simulink model "FEEDER_MODEL"  (R2024b)
settings: Solver=ode23t  StartTime=0.0  StopTime=2.4  RelTol=1e-3
libraries: spsFirstOrderFilterLib x42, spsThreePhaseVIMeasurementLib x7, spsThreePhaseDynamicLoadLib x4, spsDistributedParametersLineLib x4, spsPower3phInstantaneousLib x3, spsThreePhaseSourceLib x2, spsThreePhaseTransformerTwoWindingsLib x2, spspowerguiLib x1
(part 1 of 2)
settings Model: Creator=Baymax  LastModifiedBy=Baymax

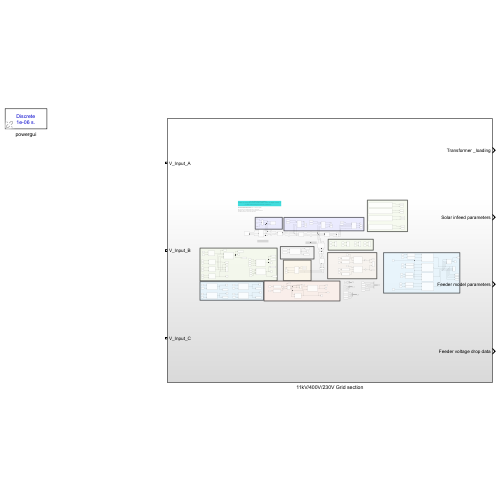
[thumbnail: Simulink's stored preview of the top-level diagram]
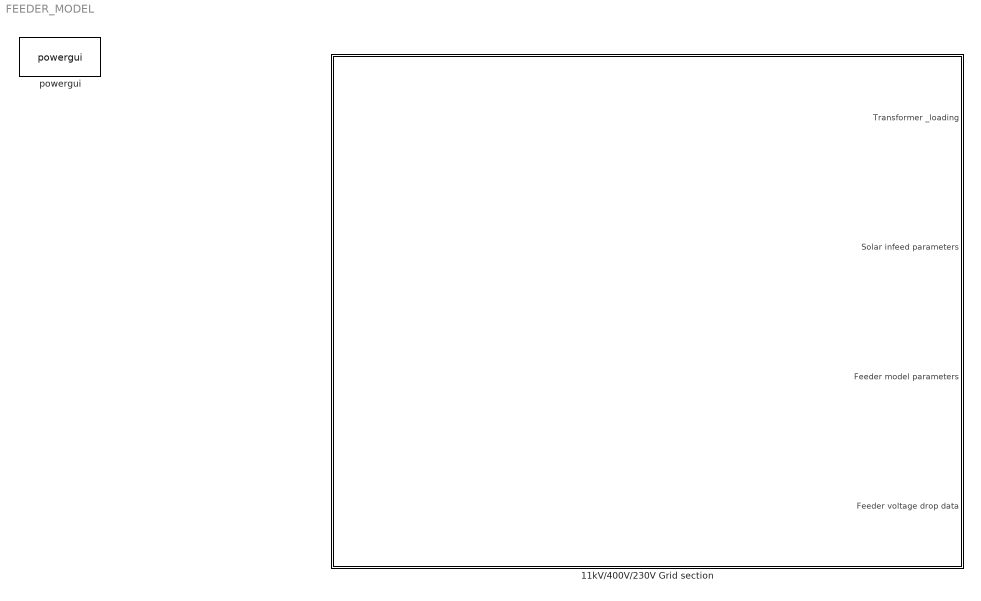
== system FEEDER_MODEL ==
  11kV/400V/230V Grid section : Subsystem
  powergui : spspowerguiLib/powergui  Priority=1  SimulationMode=Discrete  SampleTime=1e-6  frequency=60  Iterations=50  frequencyindice=50  Pbase=100e6  ErrMax=1e-4  UnitsV=kV  UnitsW=kW  buscounter=0  FunctionMessages=off  echomessages=off  EnableUseOfTLC=off  CurrentSourceSwitches=off  DisableSnubberDevices=off  DisableRonSwitches=off  DisableVfSwitches=off  DisplayEquations=off  AutomaticDiscreteSolvers=off  SolverType=Tustin/Backward Euler (TBE)  Interpol=off  ExternalGateDelay=off  methode=off  Ts=100  x0status=blocks  SPID=on  SwTol=0  HookPort=off  NonlinearTolerance=1e-4  nMaxIteration=100  ContinueOnMaxIteration=off  RestoreLinks=warning  ResistiveCurrentMeasurement=off  Frange=[0:2:500]  Ylog=off  Xlog=on  ShowGrid=off  save=off  variable=ZData  structure=0  ZoomFFT=off  StartTime=0.0  cycles=1  DisplayStyle=1  fundamental=60  FreqAxis=off  MaxFrequency=1000  frequencyindicesteady=1  RmsSteady=1  display=off

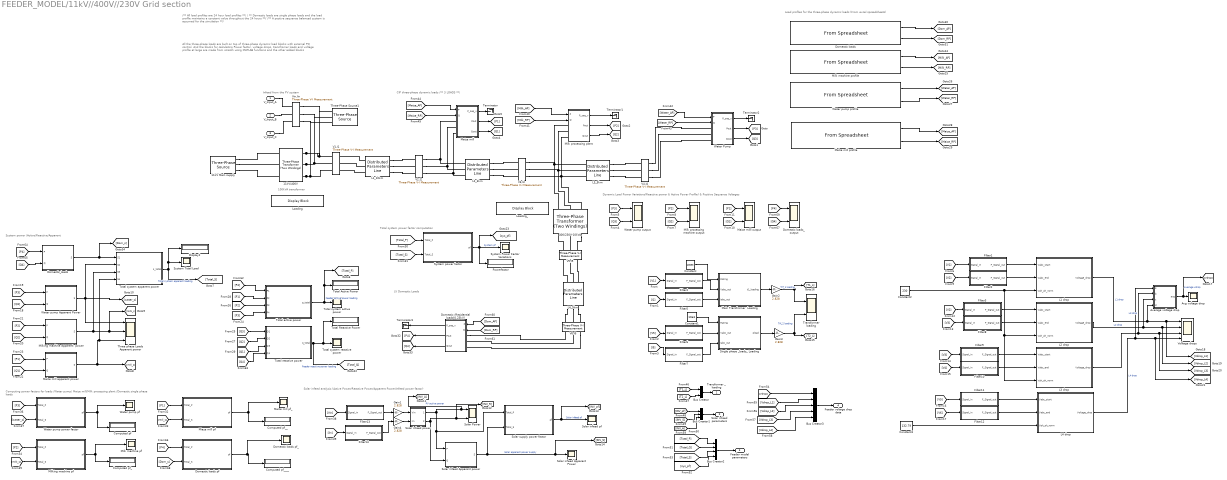
== system FEEDER_MODEL/11kV//400V//230V Grid section ==
  note: 100kVA transformer
  note: All the three-phase loads are built on top of three-phase dynamic load blocks with external PQ control.
      |
      | And the blocks for calculating Power factor, voltage drops, transfromer loads and voltage profile at large are made from scratch using MATLAB functions and the other added blocks
  note: LV Domestic Loads
  note: CIP three-phase dynamic loads /** 3 LOADS **/
  note: Solar infeed analysis (Active Power/Reactive Power/Apparent Power/Infeed power factor)
  note: Dynamic Load Power Variations(Reactive power & Active Power Profile) & Positive Sequence Voltages
  note: Computing power factors for loads /Water pump/ Maize mill/Milk processing plant /Domestic single phase loads
  note: System power /Acitve/Reactive/Apparent
  note: /** All load profiles are 24 hour load profiles **/
      |
      | / ** Domestic loads are single phase loads and the load profile maintains a constant value throughout the 24 hours **/
      |
      | /** A postive sequence balanced system is assumed for the simulation **/
  note: Load profiles for the three-phase dynamic loads (From excel spreadsheets)
  note: Total system power factor computation
  note: Infeed from the PV system
  11kV Main supply : spsThreePhaseSourceLib/Three-Phase Source  InternalConnection=Yg  VoltagePhases=off  Voltage=11e3  PhaseAngle=0  Voltage_phases=[25e3 25e3 25e3]/sqrt(3)  PhaseAngles_phases=[0 -120 +120]  Frequency=50  NonIdealSource=on  SpecifyImpedance=off  Resistance=0.8929  Inductance=16.58e-3  ShortCircuitLevel=100e6  BaseVoltage=25e3  XRratio=7  BusType=swing  Pref=10e3  Qref=0  Prefabc=[10e3, 10e3, 10e3]  Qrefabc=[0, 0, 0]  Qmin=-inf  Qmax=inf
  "11kV/400V " : spsThreePhaseTransformerTwoWindingsLib/Three-Phase Transformer (Two Windings)  Winding1Connection=Yg  Winding2Connection=Yg  CoreType=Three single-phase transformers  SetSaturation=off  Hysteresis=off  DataFile='hysteresis'  SetInitialFlux=off  Measurements=None  UNITS=pu  NominalPower=[ 100e3 , 50 ]  Winding1=[ 11e3 , 0.002 , 0.08 ]  Winding2=[ 400 , 0.002 , 0.08 ]  Rm=500  Lm=500  L0=0.5  Saturation=[ 0,0 ; 0.0024,1.2 ; 1.0,1.52 ]  InitialFluxes=[ 0.8 , -0.8 , 0.7 ]  BreakLoop=off  DiscreteSolver=Trapezoidal iterative  DataType=off  TransfoNumber=1
  "400/230V-10kVA " : spsThreePhaseTransformerTwoWindingsLib/Three-Phase Transformer (Two Windings)  Winding1Connection=Yg  Winding2Connection=Yg  CoreType=Three single-phase transformers  SetSaturation=off  Hysteresis=off  DataFile='hysteresis'  SetInitialFlux=off  Measurements=None  UNITS=pu  NominalPower=[ 10e3 , 50 ]  Winding1=[ 400 , 0.002 , 0.08 ]  Winding2=[ 230 , 0.002 , 0.08 ]  Rm=500  Lm=500  L0=0.5  Saturation=[ 0,0 ; 0.0024,1.2 ; 1.0,1.52 ]  InitialFluxes=[ 0.8 , -0.8 , 0.7 ]  BreakLoop=off  DiscreteSolver=Trapezoidal iterative  DataType=off  TransfoNumber=1
  Average voltage drop : MATLAB Function  TreatAsAtomicUnit=on
  Avg voltage drop : Scope
  Bus Creator : BusCreator  Inputs=2
  Bus Creator1 : BusCreator  Inputs=3
  Bus Creator2 : BusCreator  Inputs=4
  Bus Creator3 : BusCreator  Inputs=5
  Computed pf : Display
  Computed pf_ : Display
  Computed pf__ : Display
  Computed pf____ : Display
  Constant : Constant  Value=100e3
  Constant1 : Constant  Value=10e3
  Constant2 : Constant  Value=230
  Constant3 : Constant  Value=132.79
  Display2 : Display
  Domestic /Residential loads(0.23kV) : Subsystem
  Domestic loads : FromSpreadsheet  FileName=C:\Users\Baymax\Desktop\Mr.Usamah\Profiles\granular\h_pf\Domestic_loads.xlsx  SheetName=profile  Range=A2:C2002
  Domestic loads pf : MATLAB Function  TreatAsAtomicUnit=on
  Domestic loads pf_ : Scope
  Domestic loads_output : Scope  NumInputPorts=2
  Domestic_loads : MATLAB Function  TreatAsAtomicUnit=on
  Filter1 : Subsystem
  Filter10 : Subsystem
  Filter11 : Subsystem
  Filter12 : Subsystem
  Filter13 : Subsystem
  Filter14 : Subsystem
  Filter2 : Subsystem
  Filter3 : Subsystem
  Filter4 : Subsystem
  Filter5 : Subsystem
  Filter6 : Subsystem
  Filter7 : Subsystem
  Filter8 : Subsystem
  Filter9 : Subsystem
  Gain{1..4} (4 alike) : Gain  Gain=2.828
  L1 drop : Subsystem
  L1_10km : spsDistributedParametersLineLib/Distributed Parameters Line  Phases=3  Length=10  Frequency=50  Resistance=[0.01273 0.3864]  Inductance="[0.9337e-3  4.1264e-3]"  Capacitance=[12.74e-9 7.751e-9]  x1=[-5.7e-05 -1.52676771420257e-15 0 0;-5.6e-05 -1.49998510389932e-15 0 0;-5.5e-05 -1.47320234555348e-15 0 0;-5.4e-05 -1.44641944180839e-15 0 0;-5.3e-05 -1.41963639530743e-15 0 0;-5.2e-05 -1.39285320869397e-15 0 0;-5.1e-05 -1.36606988461142e-15 0 0;-5e-05 -1.33928642570317e-15 0 0;-4.9e-05 -1.31250283461264e-15 0 0;-4.8e-05 -1.28571911398329e-15 0 0;-4.7e-05 -1.25893526645854e-15 0 0;-4.6e-05 -1.23215129468186e-15 0 0;-4.5e-05 -1.20536720129673e-15 0 0;-4.4e-05 -1.17858298894662e-15 0 0;-4.3e-05 -1.15179866027504e-15 0 0;-4.2e-05 -1.12501421792548e-15 0 0;-4.1e-05 -1.09822966454148e-15 0 0;-4e-05 -1.07144500276655e-15 0 0;-3.9e-05 -1.04466023524424e-15 0 0;-3.8e-05 -1.01787536461809e-15 0 0;-3.7e-05 -9.91090393531678e-16 0 0;-3.6e-05 -9.64305324628563e-16 0 0;-3.5e-05 -9.37520160552329e-16 196.179007943669 -348.588291315468;-3.4e-05 -9.10734903946564e-16 196.288510502334 -348.526642661325;-3.3e-05 -8.83949557454868e-16 196.3979936881 -348.464959608981;-3.2e-05 -8.57164123720848e-16 196.507457490161 -348.403242164525;-3.1e-05 -8.30378605388121e-16 196.616901897713 -348.341490334047;-3e-05 -8.03593005100311e-16 196.726326899956 -348.279704123642;-2.9e-05 -7.76807325501051e-16 196.835732486088 -348.217883539409;-2.8e-05 -7.50021569233982e-16 196.945118645312 -348.156028587448;-2.7e-05 -7.23235738942752e-16 197.054485366832 -348.094139273865;-2.6e-05 -6.96449837271016e-16 197.163832639854 -348.032215604768;-2.5e-05 -6.69663866862436e-16 197.273160453586 -347.970257586268;-2.4e-05 -6.42877830360683e-16 197.382468797238 -347.90826522448;-2.3e-05 -6.16091730409431e-16 197.491757660021 -347.846238525524;-2.2e-05 -5.89305569652364e-16 197.601027031149 -347.78417749552;-2.1e-05 -5.62519350733168e-16 197.710276899837 -347.722082140594;-2e-05 -5.35733076295539e-16 197.819507255304 -347.659952466874;-1.9e-05 -5.08946748983174e-16 197.928718086768 -347.597788480492;-1.8e-05 -4.82160371439779e-16 198.03790938345 -347.535590187584;-1.7e-05 -4.55373946309064e-16 198.147081134575 -347.473357594289;-1.6e-05 -4.28587476234741e-16 198.256233329366 -347.411090706748;-1.5e-05 -4.01800963860531e-16 198.365365957052 -347.348789531107;-1.4e-05 -3.75014411830155e-16 198.474479006861 -347.286454073514;-1.3e-05 -3.48227822787341e-16 198.583572468024 -347.224084340123;-1.2e-05 -3.21441199375819e-16 198.692646329775 -347.161680337089;-1.1e-05 -2.94654544239322e-16 198.801700581347 -347.09924207057;-1e-05 -2.67867860021587e-16 198.910735211978 -347.03676954673;-9e-06 -2.41081149366355e-16 199.019750210907 -346.974262771734;-8e-06 -2.14294414917367e-16 199.128745567374 -346.911721751751;-7e-06 -1.87507659318368e-16 199.237721270622 -346.849146492953;-6e-06 -1.60720885213105e-16 199.346677309894 -346.786537001518;-5e-06 -1.33934095245327e-16 199.455613674439 -346.723893283623;-4e-06 -1.07147292058783e-16 199.564530353504 -346.661215345452;-3e-06 -8.03604782972257e-17 199.673427336339 -346.59850319319;-2e-06 -5.35736566044071e-17 199.782304612197 -346.535756833028;-1e-06 -2.67868296240806e-17 199.891162170332 -346.472976271158]  x2=[-5.7e-05 1.81428834656405e-11 0 0;-5.6e-05 1.81372759049777e-11 0 0;-5.5e-05 1.81316665542375e-11 0 0;-5.4e-05 1.81260554139736e-11 0 0;-5.3e-05 1.81204424847397e-11 0 0;-5.2e-05 1.81148277670899e-11 0 0;-5.1e-05 1.81092112615782e-11 0 0;-5e-05 1.81035929687591e-11 0 0;-4.9e-05 1.80979728891869e-11 0 0;-4.8e-05 1.80923510234165e-11 0 0;-4.7e-05 1.80867273720025e-11 0 0;-4.6e-05 1.80811019355002e-11 0 0;-4.5e-05 1.80754747144646e-11 0 0;-4.4e-05 1.80698457094512e-11 0 0;-4.3e-05 1.80642149210156e-11 0 0;-4.2e-05 1.80585823497133e-11 0 0;-4.1e-05 1.80529479961005e-11 0 0;-4e-05 1.80473118607331e-11 0 0;-3.9e-05 1.80416739441675e-11 0 0;-3.8e-05 1.803603424696e-11 0 0;-3.7e-05 1.80303927696673e-11 0 0;-3.6e-05 1.80247495128462e-11 0 0;-3.5e-05 1.80191044770537e-11 100.365229967348 -319.80964811604;-3.4e-05 1.80134576628468e-11 100.465696176977 -319.778101667671;-3.3e-05 1.80078090707829e-11 100.566152471039 -319.746523658469;-3.2e-05 1.80021587014195e-11 100.66659883962 -319.71491409155;-3.1e-05 1.79965065553143e-11 100.767035272805 -319.683272970034;-3e-05 1.79908526330251e-11 100.867461760683 -319.651600297044;-2.9e-05 1.798519693511e-11 100.967878293342 -319.619896075706;-2.8e-05 1.7979539462127e-11 101.06828486087 -319.588160309149;-2.7e-05 1.79738802146347e-11 101.168681453359 -319.556393000505;-2.6e-05 1.79682191931915e-11 101.269068060899 -319.524594152909;-2.5e-05 1.79625563983561e-11 101.369444673583 -319.4927637695;-2.4e-05 1.79568918306875e-11 101.469811281504 -319.46090185342;-2.3e-05 1.79512254907448e-11 101.570167874756 -319.429008407812;-2.2e-05 1.79455573790871e-11 101.670514443434 -319.397083435826;-2.1e-05 1.79398874962739e-11 101.770850977634 -319.365126940611;-2e-05 1.79342158428648e-11 101.871177467455 -319.333138925321;-1.9e-05 1.79285424194196e-11 101.971493902993 -319.301119393115;-1.8e-05 1.79228672264981e-11 102.071800274348 -319.269068347151;-1.7e-05 1.79171902646606e-11 102.172096571621 -319.236985790593;-1.6e-05 1.79115115344673e-11 102.272382784912 -319.204871726609;-1.5e-05 1.79058310364787e-11 102.372658904323 -319.172726158366;-1.4e-05 1.79001487712554e-11 102.472924919958 -319.140549089038;-1.3e-05 1.78944647393583e-11 102.573180821921 -319.108340521801;-1.2e-05 1.78887789413483e-11 102.673426600316 -319.076100459833;-1.1e-05 1.78830913777865e-11 102.773662245251 -319.043828906317;-1e-05 1.78774020492345e-11 102.873887746832 -319.011525864437;-9e-06 1.78717109562536e-11 102.974103095167 -318.979191337382;-8e-06 1.78660180994055e-11 103.074308280366 -318.946825328343;-7e-06 1.78603234792521e-11 103.174503292538 -318.914427840514;-6e-06 1.78546270963555e-11 103.274688121795 -318.881998877093;-5e-06 1.78489289512778e-11 103.374862758249 -318.84953844128;-4e-06 1.78432290445815e-11 103.475027192013 -318.81704653628;-3e-06 1.78375273768291e-11 103.575181413202 -318.784523165298;-2e-06 1.78318239485833e-11 103.675325411929 -318.751968331546;-1e-06 1.7826118760407e-11 103.775459178313 -318.719382038235]  x3=[-5.7e-05 1.64428180664199e-12 0 0;-5.6e-05 1.6445629111865e-12 0 0;-5.5e-05 1.64484385341915e-12 0 0;-5.4e-05 1.64512463331223e-12 0 0;-5.3e-05 1.64540525083801e-12 0 0;-5.2e-05 1.6456857059688e-12 0 0;-5.1e-05 1.64596599867693e-12 0 0;-5e-05 1.64624612893472e-12 0 0;-4.9e-05 1.64652609671454e-12 0 0;-4.8e-05 1.64680590198874e-12 0 0;-4.7e-05 1.64708554472972e-12 0 0;-4.6e-05 1.64736502490987e-12 0 0;-4.5e-05 1.64764434250162e-12 0 0;-4.4e-05 1.64792349747738e-12 0 0;-4.3e-05 1.64820248980962e-12 0 0;-4.2e-05 1.64848131947079e-12 0 0;-4.1e-05 1.64875998643338e-12 0 0;-4e-05 1.64903849066988e-12 0 0;-3.9e-05 1.64931683215281e-12 0 0;-3.8e-05 1.6495950108547e-12 0 0;-3.7e-05 1.64987302674808e-12 0 0;-3.6e-05 1.65015087980552e-12 0 0;-3.5e-05 1.6504285699996e-12 9.09331411230753 31.7294413538396;-3.4e-05 1.65070609730291e-12 9.08334556574846 31.7322965368886;-3.3e-05 1.65098346168806e-12 9.07337612269913 31.7351485880856;-3.2e-05 1.65126066312768e-12 9.06340578414348 31.7379975071489;-3.1e-05 1.6515377015944e-12 9.05343455106554 31.7408432937975;-3e-05 1.65181457706089e-12 9.04346242444943 31.7436859477504;-2.9e-05 1.65209128949981e-12 9.03348940527936 31.7465254687272;-2.8e-05 1.65236783888386e-12 9.02351549453963 31.7493618564474;-2.7e-05 1.65264422518574e-12 9.01354069321463 31.7521951106313;-2.6e-05 1.65292044837818e-12 9.00356500228882 31.7550252309992;-2.5e-05 1.65319650843391e-12 8.99358842274678 31.7578522172717;-2.4e-05 1.65347240532568e-12 8.98361095557314 31.7606760691699;-2.3e-05 1.65374813902627e-12 8.97363260175265 31.763496786415;-2.2e-05 1.65402370950846e-12 8.96365336227012 31.7663143687287;-2.1e-05 1.65429911674506e-12 8.95367323811048 31.7691288158328;-2e-05 1.65457436070888e-12 8.94369223025872 31.7719401274497;-1.9e-05 1.65484944137276e-12 8.93371033969992 31.7747483033017;-1.8e-05 1.65512435870954e-12 8.92372756741926 31.7775533431118;-1.7e-05 1.6553991126921e-12 8.913743914402 31.7803552466032;-1.6e-05 1.65567370329332e-12 8.90375938163348 31.7831540134992;-1.5e-05 1.65594813048609e-12 8.89377397009915 31.7859496435237;-1.4e-05 1.65622239424334e-12 8.88378768078451 31.7887421364007;-1.3e-05 1.65649649453799e-12 8.87380051467519 31.7915314918547;-1.2e-05 1.65677043134299e-12 8.86381247275686 31.7943177096102;-1.1e-05 1.6570442046313e-12 8.85382355601531 31.7971007893925;-1e-05 1.65731781437591e-12 8.84383376543641 31.7998807309267;-9e-06 1.65759126054981e-12 8.83384310200612 31.8026575339385;-8e-06 1.657864543126e-12 8.82385156671046 31.8054311981538;-7e-06 1.65813766207753e-12 8.81385916053556 31.808201723299;-6e-06 1.65841061737743e-12 8.80386588446765 31.8109691091004;-5e-06 1.65868340899877e-12 8.793871739493 31.8137333552851;-4e-06 1.65895603691461e-12 8.78387672659801 31.8164944615802;-3e-06 1.65922850109806e-12 8.77388084676914 31.8192524277132;-2e-06 1.65950080152222e-12 8.76388410099295 31.8220072534119;-1e-06 1.65977293816022e-12 8.75388649025608 31.8247589384044]  x4=[-5.7e-05 -1.63484597482052e-12 0 0;-5.6e-05 -1.63513718601473e-12 0 0;-5.5e-05 -1.63542823582736e-12 0 0;-5.4e-05 -1.6357191242297e-12 0 0;-5.3e-05 -1.63600985119304e-12 0 0;-5.2e-05 -1.63630041668867e-12 0 0;-5.1e-05 -1.63659082068793e-12 0 0;-5e-05 -1.63688106316215e-12 0 0;-4.9e-05 -1.63717114408269e-12 0 0;-4.8e-05 -1.63746106342091e-12 0 0;-4.7e-05 -1.6377508211482e-12 0 0;-4.6e-05 -1.63804041723597e-12 0 0;-4.5e-05 -1.63832985165563e-12 0 0;-4.4e-05 -1.63861912437862e-12 0 0;-4.3e-05 -1.63890823537638e-12 0 0;-4.2e-05 -1.63919718462038e-12 0 0;-4.1e-05 -1.63948597208211e-12 0 0;-4e-05 -1.63977459773306e-12 0 0;-3.9e-05 -1.64006306154475e-12 0 0;-3.8e-05 -1.6403513634887e-12 0 0;-3.7e-05 -1.64063950353646e-12 0 0;-3.6e-05 -1.6409274816596e-12 0 0;-3.5e-05 -1.64121529782968e-12 -8.01167886415262 -34.2034757112838;-3.4e-05 -1.64150295201831e-12 -8.00093313016669 -34.2059909665148;-3.3e-05 -1.64179044419709e-12 -7.99018660652032 -34.2085028457499;-3.2e-05 -1.64207777433766e-12 -7.97943929427415 -34.211011348741;-3.1e-05 -1.64236494241164e-12 -7.96869119448889 -34.2135164752407;-3e-05 -1.6426519483907e-12 -7.95794230822534 -34.2160182250017;-2.9e-05 -1.64293879224652e-12 -7.94719263654438 -34.2185165977771;-2.8e-05 -1.64322547395077e-12 -7.93644218050694 -34.2210115933203;-2.7e-05 -1.64351199347518e-12 -7.92569094117407 -34.2235032113851;-2.6e-05 -1.64379835079145e-12 -7.91493891960686 -34.2259914517255;-2.5e-05 -1.64408454587133e-12 -7.9041861168665 -34.228476314096;-2.4e-05 -1.64437057868657e-12 -7.89343253401424 -34.2309577982513;-2.3e-05 -1.64465644920894e-12 -7.88267817211142 -34.2334359039465;-2.2e-05 -1.64494215741023e-12 -7.87192303221946 -34.235910630937;-2.1e-05 -1.64522770326223e-12 -7.86116711539984 -34.2383819789786;-2e-05 -1.64551308673678e-12 -7.85041042271414 -34.2408499478274;-1.9e-05 -1.64579830780569e-12 -7.83965295522399 -34.2433145372398;-1.8e-05 -1.64608336644081e-12 -7.82889471399111 -34.2457757469726;-1.7e-05 -1.64636826261403e-12 -7.8181357000773 -34.2482335767828;-1.6e-05 -1.64665299629721e-12 -7.80737591454443 -34.2506880264278;-1.5e-05 -1.64693756746225e-12 -7.79661535845445 -34.2531390956654;-1.4e-05 -1.64722197608108e-12 -7.78585403286938 -34.2555867842538;-1.3e-05 -1.64750622212561e-12 -7.77509193885133 -34.2580310919513;-1.2e-05 -1.6477903055678e-12 -7.76432907746247 -34.2604720185167;-1.1e-05 -1.6480742263796e-12 -7.75356544976505 -34.262909563709;-1e-05 -1.648357984533e-12 -7.7428010568214 -34.2653437272877;-9e-06 -1.64864157999999e-12 -7.73203589969392 -34.2677745090126;-8e-06 -1.64892501275258e-12 -7.7212699794451 -34.2702019086438;-7e-06 -1.64920828276279e-12 -7.71050329713747 -34.2726259259416;-6e-06 -1.64949139000267e-12 -7.69973585383369 -34.2750465606669;-5e-06 -1.64977433444428e-12 -7.68896765059643 -34.2774638125806;-4e-06 -1.65005711605969e-12 -7.6781986884885 -34.2798776814443;-3e-06 -1.65033973482099e-12 -7.66742896857274 -34.2822881670198;-2e-06 -1.65062219070029e-12 -7.65665849191207 -34.284695269069;-1e-06 -1.65090448366971e-12 -7.64588725956951 -34.2870989873545]  x5=5.65541566995743e-05  V1=ones(3,3)  V2=ones(3,3)  I1=ones(3,3)  I2=ones(3,3)  nHarmo=1  Measurements=None  Decoupling=off  VsMag0=0  VrMag0=0  VsAngle0=0  VrAngle0=0  IsMag0=0  IrMag0=0  IsAngle0=0  IrAngle0=0
      settings: LibrarySourceBlock=sps_lib/Power Grid Elements/Distributed Parameters Line
  L2 drop : Subsystem
  L2_3km : spsDistributedParametersLineLib/Distributed Parameters Line  Phases=3  Length=3  Frequency=50  Resistance=[0.01273 0.3864]  Inductance="[0.9337e-3  4.1264e-3]"  Capacitance=[12.74e-9 7.751e-9]  x1=[-1.7e-05 1.79172282124895e-11 0 0;-1.6e-05 1.79115472500903e-11 0 0;-1.5e-05 1.79058645198924e-11 0 0;-1.4e-05 1.79001800224564e-11 0 0;-1.3e-05 1.78944937583435e-11 0 0;-1.2e-05 1.78888057281149e-11 0 0;-1.1e-05 1.78831159323319e-11 102.773662245251 -319.043828906317;-1e-05 1.78774243715561e-11 102.873887746832 -319.011525864437;-9e-06 1.78717310463493e-11 102.974103095167 -318.979191337382;-8e-06 1.78660359572734e-11 103.074308280366 -318.946825328343;-7e-06 1.78603391048904e-11 103.174503292538 -318.914427840514;-6e-06 1.78546404897626e-11 103.274688121795 -318.881998877093;-5e-06 1.78489401124524e-11 103.374862758249 -318.84953844128;-4e-06 1.78432379735225e-11 103.475027192013 -318.81704653628;-3e-06 1.78375340735356e-11 103.575181413202 -318.784523165298;-2e-06 1.78318284130546e-11 103.675325411929 -318.751968331546;-1e-06 1.78261209926428e-11 103.775459178313 -318.719382038235]  x2=[-1.7e-05 2.09734489341479e-11 0 0;-1.6e-05 2.09668822740188e-11 0 0;-1.5e-05 2.09603135445414e-11 0 0;-1.4e-05 2.0953742746364e-11 0 0;-1.3e-05 2.0947169880135e-11 0 0;-1.2e-05 2.09405949465033e-11 0 0;-1.1e-05 2.09340179461177e-11 76.4647485589338 -311.350409441593;-1e-05 2.09274388796274e-11 76.5625583998402 -311.326371968229;-9e-06 2.09208577476817e-11 76.660360684325 -311.302303768183;-8e-06 2.09142745509301e-11 76.7581554027355 -311.278204843832;-7e-06 2.09076892900223e-11 76.8559425454198 -311.254075197553;-6e-06 2.09011019656084e-11 76.9537221027266 -311.229914831729;-5e-06 2.08945125783383e-11 77.0514940650056 -311.205723748743;-4e-06 2.08879211288626e-11 77.149258422607 -311.181501950985;-3e-06 2.08813276178317e-11 77.2470151658819 -311.157249440843;-2e-06 2.08747320458964e-11 77.344764285182 -311.132966220712;-1e-06 2.08681344137076e-11 77.4425057708599 -311.108652292988]  x3=[-1.7e-05 8.6696225978401e-13 0 0;-1.6e-05 8.67125382527385e-13 0 0;-1.5e-05 8.67288419688916e-13 0 0;-1.4e-05 8.67451371252512e-13 0 0;-1.3e-05 8.6761423720209e-13 0 0;-1.2e-05 8.67777017521575e-13 0 0;-1.1e-05 8.67939712194903e-13 7.8083141716271 29.038202858794;-1e-05 8.68102321206015e-13 7.79919116597484 29.0406544800196;-9e-06 8.68264844538863e-13 7.79006739057327 29.0431032350476;-8e-06 8.68427282177406e-13 7.78094284632288 29.0455491236362;-7e-06 8.68589634105613e-13 7.77181753412421 29.047992145544;-6e-06 8.6875190030746e-13 7.7626914548779 29.0504323005299;-5e-06 8.68914080766931e-13 7.75356460948467 29.0528695883531;-4e-06 8.69076175468021e-13 7.74443699884528 29.055304008773;-3e-06 8.69238184394731e-13 7.73530862386061 29.0577355615494;-2e-06 8.69400107531072e-13 7.72617948543158 29.0601642464423;-1e-06 8.69561944861063e-13 7.71704958445921 29.0625900632119]  x4=[-1.7e-05 -8.91545729988945e-13 0 0;-1.6e-05 -8.9172450623222e-13 0 0;-1.5e-05 -8.91903194465814e-13 0 0;-1.4e-05 -8.92081794672092e-13 0 0;-1.3e-05 -8.92260306833426e-13 0 0;-1.2e-05 -8.92438730932199e-13 0 0;-1.1e-05 -8.926170669508e-13 -7.1500860619961 -31.3676237981618;-1e-05 -8.92795314871629e-13 -7.14023127966711 -31.3698685159791;-9e-06 -8.92973474677092e-13 -7.13037579262555 -31.3721101377146;-8e-06 -8.93151546349607e-13 -7.1205196018441 -31.3743486631469;-7e-06 -8.93329529871599e-13 -7.11066270829555 -31.3765840920552;-6e-06 -8.935074252255e-13 -7.10080511295272 -31.3788164242187;-5e-06 -8.93685232393754e-13 -7.09094681678853 -31.3810456594173;-4e-06 -8.93862951358812e-13 -7.08108782077594 -31.3832717974308;-3e-06 -8.94040582103133e-13 -7.071228125888 -31.3854948380395;-2e-06 -8.94218124609187e-13 -7.06136773309783 -31.3877147810241;-1e-06 -8.9439557885945e-13 -7.0515066433786 -31.3899316261655]  x5=1.69662470098723e-05  V1=ones(3,3)  V2=ones(3,3)  I1=ones(3,3)  I2=ones(3,3)  nHarmo=1  Measurements=None  Decoupling=off  VsMag0=0  VrMag0=0  VsAngle0=0  VrAngle0=0  IsMag0=0  IrMag0=0  IsAngle0=0  IrAngle0=0
      settings: LibrarySourceBlock=sps_lib/Power Grid Elements/Distributed Parameters Line
  L3 drop : Subsystem
  L3_5km : spsDistributedParametersLineLib/Distributed Parameters Line  Phases=3  Length=5  Frequency=50  Resistance=[0.01273 0.3864]  Inductance="[0.9337e-3  4.1264e-3]"  Capacitance=[12.74e-9 7.751e-9]  x1=[-2.9e-05 2.10520224768795e-11 0 0;-2.8e-05 2.10454829315702e-11 0 0;-2.7e-05 2.10389413091549e-11 0 0;-2.6e-05 2.10323976102794e-11 0 0;-2.5e-05 2.10258518355895e-11 0 0;-2.4e-05 2.10193039857312e-11 0 0;-2.3e-05 2.10127540613508e-11 0 0;-2.2e-05 2.10062020630947e-11 0 0;-2.1e-05 2.09996479916096e-11 0 0;-2e-05 2.09930918475423e-11 0 0;-1.9e-05 2.09865336315399e-11 0 0;-1.8e-05 2.09799733442496e-11 75.7798689037684 -311.517811209177;-1.7e-05 2.09734109863191e-11 75.8777313692877 -311.493988888837;-1.6e-05 2.09668465583958e-11 75.9755863459751 -311.470135825273;-1.5e-05 2.09602800611277e-11 76.0734338241727 -311.446252020839;-1.4e-05 2.0953711495163e-11 76.1712737942235 -311.422337477892;-1.3e-05 2.09471408611498e-11 76.2691062464709 -311.398392198793;-1.2e-05 2.09405681597367e-11 76.3669311712593 -311.374416185905;-1.1e-05 2.09339933915724e-11 76.4647485589338 -311.350409441593;-1e-05 2.09274165573057e-11 76.5625583998402 -311.326371968229;-9e-06 2.09208376575859e-11 76.660360684325 -311.302303768183;-8e-06 2.09142566930622e-11 76.7581554027355 -311.278204843832;-7e-06 2.0907673664384e-11 76.8559425454198 -311.254075197553;-6e-06 2.09010885722013e-11 76.9537221027266 -311.229914831729;-5e-06 2.08945014171637e-11 77.0514940650056 -311.205723748743;-4e-06 2.08879121999216e-11 77.149258422607 -311.181501950985;-3e-06 2.08813209211252e-11 77.2470151658819 -311.157249440843;-2e-06 2.0874727581425e-11 77.344764285182 -311.132966220712;-1e-06 2.08681321814718e-11 77.4425057708599 -311.108652292988]  x2=[-2.9e-05 2.41436411191213e-11 0 0;-2.8e-05 2.41353645894314e-11 0 0;-2.7e-05 2.41270856776764e-11 0 0;-2.6e-05 2.41188043846736e-11 0 0;-2.5e-05 2.41105207112403e-11 0 0;-2.4e-05 2.41022346581939e-11 0 0;-2.3e-05 2.40939462263524e-11 0 0;-2.2e-05 2.40856554165337e-11 0 0;-2.1e-05 2.40773622295561e-11 0 0;-2e-05 2.40690666662381e-11 0 0;-1.9e-05 2.40607687273985e-11 0 0;-1.8e-05 2.40524684138563e-11 73.6970709105077 -310.908849021923;-1.7e-05 2.40441657264305e-11 73.7947421676987 -310.88568106191;-1.6e-05 2.40358606659407e-11 73.8924061416407 -310.862482418712;-1.5e-05 2.40275532332066e-11 73.9900628226945 -310.839253094616;-1.4e-05 2.40192434290481e-11 74.0877122012219 -310.815993091916;-1.3e-05 2.40109312542853e-11 74.1853542675852 -310.792702412907;-1.2e-05 2.40026167097385e-11 74.2829890121476 -310.769381059889;-1.1e-05 2.39942997962285e-11 74.380616425273 -310.746029035162;-1e-05 2.3985980514576e-11 74.4782364973258 -310.722646341031;-9e-06 2.39776588656022e-11 74.5758492186713 -310.699232979805;-8e-06 2.39693348501283e-11 74.6734545796756 -310.675788953794;-7e-06 2.39610084689759e-11 74.7710525707054 -310.652314265312;-6e-06 2.39526797229667e-11 74.8686431821282 -310.628808916675;-5e-06 2.39443486129229e-11 74.9662264043121 -310.605272910204;-4e-06 2.39360151396666e-11 75.0638022276262 -310.581706248222;-3e-06 2.39276793040203e-11 75.1613706424399 -310.558108933054;-2e-06 2.39193411068067e-11 75.2589316391238 -310.53448096703;-1e-06 2.39110005488488e-11 75.3564852080489 -310.510822352481]  x3=[-2.9e-05 9.34561060055704e-13 0 0;-2.8e-05 9.34615190941869e-13 0 0;-2.7e-05 9.34669229585212e-13 0 0;-2.6e-05 9.34723175980401e-13 0 0;-2.5e-05 9.34777030122111e-13 0 0;-2.4e-05 9.34830792005027e-13 0 0;-2.3e-05 9.34884461623842e-13 0 0;-2.2e-05 9.3493803897326e-13 0 0;-2.1e-05 9.34991524047993e-13 0 0;-2e-05 9.35044916842763e-13 0 0;-1.9e-05 9.35098217352299e-13 0 0;-1.8e-05 9.3515142557134e-13 0.629626177120523 0.283997051848631;-1.7e-05 9.35204541494637e-13 0.629536925746012 0.284194840727939;-1.6e-05 9.35257565116945e-13 0.629447612238697 0.284392601558341;-1.5e-05 9.35310496433032e-13 0.629358236607393 0.284590334320318;-1.4e-05 9.35363335437675e-13 0.629268798860922 0.284788038994355;-1.3e-05 9.35416082125657e-13 0.62917929900811 0.28498571556094;-1.2e-05 9.35468736491773e-13 0.629089737057791 0.285183364000562;-1.1e-05 9.35521298530826e-13 0.629000113018804 0.285380984293715;-1e-05 9.35573768237629e-13 0.628910426899995 0.285578576420893;-9e-06 9.35626145607002e-13 0.628820678710215 0.285776140362597;-8e-06 9.35678430633777e-13 0.628730868458322 0.285973676099325;-7e-06 9.35730623312794e-13 0.628640996153181 0.286171183611584;-6e-06 9.357827236389e-13 0.62855106180366 0.286368662879879;-5e-06 9.35834731606954e-13 0.628461065418637 0.28656611388472;-4e-06 9.35886647211823e-13 0.628371007006993 0.28676353660662;-3e-06 9.35938470448384e-13 0.628280886577617 0.286960931026093;-2e-06 9.3599020131152e-13 0.628190704139403 0.287158297123658;-1e-06 9.36041839796127e-13 0.628100459701253 0.287355634879835]  x4=[-2.9e-05 -9.15844891850392e-13 0 0;-2.8e-05 -9.15914495160389e-13 0 0;-2.7e-05 -9.15984008073248e-13 0 0;-2.6e-05 -9.16053430582111e-13 0 0;-2.5e-05 -9.16122762680125e-13 0 0;-2.4e-05 -9.16192004360447e-13 0 0;-2.3e-05 -9.16261155616243e-13 0 0;-2.2e-05 -9.16330216440689e-13 0 0;-2.1e-05 -9.16399186826969e-13 0 0;-2e-05 -9.16468066768274e-13 0 0;-1.9e-05 -9.16536856257807e-13 0 0;-1.8e-05 -9.1660555528878e-13 -0.0838031426405297 -2.58424729295615;-1.7e-05 -9.16674163854411e-13 -0.0829912732873043 -2.58427349296195;-1.6e-05 -9.16742681947929e-13 -0.0821793957431687 -2.58429943791019;-1.5e-05 -9.16811109562572e-13 -0.0813675100882518 -2.58432512779829;-1.4e-05 -9.16879446691585e-13 -0.0805556164026836 -2.58435056262373;-1.3e-05 -9.16947693328226e-13 -0.0797437147665949 -2.584375742384;-1.2e-05 -9.17015849465757e-13 -0.078931805260117 -2.5844006670766;-1.1e-05 -9.17083915097452e-13 -0.0781198879633823 -2.58442533669909;-1e-05 -9.17151890216594e-13 -0.0773079629565238 -2.58444975124902;-9e-06 -9.17219774816473e-13 -0.0764960303196751 -2.58447391072399;-8e-06 -9.17287568890389e-13 -0.075684090132971 -2.5844978151216;-7e-06 -9.17355272431652e-13 -0.0748721424765467 -2.58452146443951;-6e-06 -9.1742288543358e-13 -0.0740601874305381 -2.58454485867538;-5e-06 -9.17490407889498e-13 -0.0732482250750821 -2.5845679978269;-4e-06 -9.17557839792744e-13 -0.0724362554903161 -2.58459088189178;-3e-06 -9.17625181136662e-13 -0.0716242787563783 -2.58461351086777;-2e-06 -9.17692431914605e-13 -0.0708122949534075 -2.58463588475263;-1e-06 -9.17759592119935e-13 -0.0700003041615435 -2.58465800354416]  x5=2.82770783497871e-05  V1=ones(3,3)  V2=ones(3,3)  I1=ones(3,3)  I2=ones(3,3)  nHarmo=1  Measurements=None  Decoupling=off  VsMag0=0  VrMag0=0  VsAngle0=0  VrAngle0=0  IsMag0=0  IrMag0=0  IsAngle0=0  IrAngle0=0
      settings: LibrarySourceBlock=sps_lib/Power Grid Elements/Distributed Parameters Line
  L4 drop : Subsystem
  L4_5km : spsDistributedParametersLineLib/Distributed Parameters Line  Phases=3  Length=5  Frequency=50  Resistance=[0.01273 0.3864]  Inductance="[0.9337e-3  4.1264e-3]"  Capacitance=[12.74e-9 7.751e-9]  x1=[-2.9e-05 5.84567014245037e-11 0 0;-2.8e-05 5.84538298916303e-11 0 0;-2.7e-05 5.84509525895951e-11 0 0;-2.6e-05 5.84480695186823e-11 0 0;-2.5e-05 5.84451806791761e-11 0 0;-2.4e-05 5.8442286071362e-11 0 0;-2.3e-05 5.84393856955254e-11 0 0;-2.2e-05 5.84364795519527e-11 0 0;-2.1e-05 5.84335676409307e-11 0 0;-2e-05 5.84306499627468e-11 0 0;-1.9e-05 5.84277265176889e-11 0 0;-1.8e-05 5.84247973060457e-11 161.37609514 67.1537265328749;-1.7e-05 5.8421862328106e-11 161.397184141456 67.1030254243096;-1.6e-05 5.84189215841598e-11 161.418257213648 67.0523176929412;-1.5e-05 5.84159750744971e-11 161.439314354497 67.0016033437744;-1.4e-05 5.84130227994088e-11 161.460355561924 66.9508823818144;-1.3e-05 5.84100647591864e-11 161.481380833853 66.9001548120673;-1.2e-05 5.84071009541216e-11 161.502390168209 66.8494206395395;-1.1e-05 5.84041313845071e-11 161.523383562918 66.7986798692385;-1e-05 5.84011560506359e-11 161.544361015908 66.7479325061721;-9e-06 5.83981749528017e-11 161.565322525108 66.6971785553488;-8e-06 5.83951880912987e-11 161.586268088451 66.6464180217779;-7e-06 5.83921954664216e-11 161.607197703869 66.5956509104693;-6e-06 5.8389197078466e-11 161.628111369295 66.5448772264334;-5e-06 5.83861929277276e-11 161.649009082666 66.4940969746815;-4e-06 5.8383183014503e-11 161.66989084192 66.4433101602253;-3e-06 5.83801673390892e-11 161.690756644996 66.3925167880772;-2e-06 5.8377145901784e-11 161.711606489833 66.3417168632505;-1e-06 5.83741187028854e-11 161.732440374375 66.2909103907588]  x2=[-2.9e-05 6.24517770249178e-11 0 0;-2.8e-05 6.24490930838053e-11 0 0;-2.7e-05 6.24464029792145e-11 0 0;-2.6e-05 6.24437067114107e-11 0 0;-2.5e-05 6.24410042806602e-11 0 0;-2.4e-05 6.24382956872297e-11 0 0;-2.3e-05 6.24355809313864e-11 0 0;-2.2e-05 6.24328600133983e-11 0 0;-2.1e-05 6.24301329335339e-11 0 0;-2e-05 6.24273996920625e-11 0 0;-1.9e-05 6.24246602892537e-11 0 0;-1.8e-05 6.2421914725378e-11 134.017837166134 93.2027487562525;-1.7e-05 6.24191630007063e-11 134.047111059216 93.1606412123047;-1.6e-05 6.24164051155101e-11 134.076371722379 93.1185244737702;-1.5e-05 6.24136410700618e-11 134.105619152734 93.0763985448058;-1.4e-05 6.2410870864634e-11 134.134853347395 93.0342634295692;-1.3e-05 6.24080944995002e-11 134.164074303477 92.9921191322188;-1.2e-05 6.24053119749345e-11 134.193282018095 92.9499656569143;-1.1e-05 6.24025232912113e-11 134.222476488368 92.9078030078159;-1e-05 6.2399728448606e-11 134.251657711413 92.865631189085;-9e-06 6.23969274473945e-11 134.280825684351 92.8234502048837;-8e-06 6.23941202878531e-11 134.309980404302 92.7812600593752;-7e-06 6.23913069702589e-11 134.33912186839 92.7390607567234;-6e-06 6.23884874948895e-11 134.368250073739 92.6968523010933;-5e-06 6.23856618620234e-11 134.397365017472 92.6546346966507;-4e-06 6.23828300719392e-11 134.426466696718 92.6124079475622;-3e-06 6.23799921249165e-11 134.455555108603 92.5701720579955;-2e-06 6.23771480212355e-11 134.484630250257 92.5279270321191;-1e-06 6.23742977611767e-11 134.51369211881 92.4856728741024]  x3=[-2.9e-05 1.57949159224884e-13 0 0;-2.8e-05 1.58130740234848e-13 0 0;-2.7e-05 1.58312305637934e-13 0 0;-2.6e-05 1.58493855416222e-13 0 0;-2.5e-05 1.58675389551794e-13 0 0;-2.4e-05 1.58856908026732e-13 0 0;-2.3e-05 1.59038410823122e-13 0 0;-2.2e-05 1.5921989792305e-13 0 0;-2.1e-05 1.59401369308605e-13 0 0;-2e-05 1.59582824961874e-13 0 0;-1.9e-05 1.59764264864951e-13 0 0;-1.8e-05 1.59945688999927e-13 -17.9380699018709 -17.5974981800289;-1.7e-05 1.60127097348896e-13 -17.9435974336721 -17.5918619008575;-1.6e-05 1.60308489893954e-13 -17.9491231945112 -17.586223885439;-1.5e-05 1.60489866617198e-13 -17.9546471838429 -17.5805841343298;-1.4e-05 1.60671227500728e-13 -17.960169401122 -17.5749426480864;-1.3e-05 1.60852572526643e-13 -17.9656898458034 -17.5692994272658;-1.2e-05 1.61033901677046e-13 -17.9712085173423 -17.5636544724249;-1.1e-05 1.6121521493404e-13 -17.976725415194 -17.5580077841207;-1e-05 1.6139651227973e-13 -17.982240538814 -17.5523593629107;-9e-06 1.61577793696223e-13 -17.9877538876581 -17.5467092093522;-8e-06 1.61759059165627e-13 -17.993265461182 -17.541057324003;-7e-06 1.61940308670052e-13 -17.9987752588419 -17.5354037074208;-6e-06 1.62121542191609e-13 -18.0042832800938 -17.5297483601636;-5e-06 1.62302759712412e-13 -18.0097895243942 -17.5240912827897;-4e-06 1.62483961214574e-13 -18.0152939911996 -17.5184324758573;-3e-06 1.62665146680212e-13 -18.0207966799669 -17.5127719399249;-2e-06 1.62846316091444e-13 -18.0262975901527 -17.5071096755512;-1e-06 1.63027469430389e-13 -18.0317967212144 -17.5014456832951]  x4=[-2.9e-05 -1.58567387636513e-14 0 0;-2.8e-05 -1.60440508605435e-14 0 0;-2.7e-05 -1.62313613739514e-14 0 0;-2.6e-05 -1.64186702853881e-14 0 0;-2.5e-05 -1.6605977576367e-14 0 0;-2.4e-05 -1.67932832284017e-14 0 0;-2.3e-05 -1.69805872230057e-14 0 0;-2.2e-05 -1.7167889541693e-14 0 0;-2.1e-05 -1.73551901659775e-14 0 0;-2e-05 -1.75424890773734e-14 0 0;-1.9e-05 -1.77297862573951e-14 0 0;-1.8e-05 -1.7917081687557e-14 19.0274185208043 18.1926842960287;-1.7e-05 -1.81043753493738e-14 19.0331329820782 18.1867057585299;-1.6e-05 -1.82916672243604e-14 19.0388455648572 18.1807254260752;-1.5e-05 -1.84789572940319e-14 19.0445562685774 18.1747432992548;-1.4e-05 -1.86662455399033e-14 19.0502650926753 18.1687593786592;-1.3e-05 -1.88535319434902e-14 19.0559720365874 18.1627736648789;-1.2e-05 -1.90408164863081e-14 19.0616770997504 18.1567861585047;-1.1e-05 -1.92280991498728e-14 19.0673802816014 18.1507968601275;-1e-05 -1.94153799157001e-14 19.0730815815774 18.1448057703386;-9e-06 -1.96026587653063e-14 19.0787809991156 18.1388128897291;-8e-06 -1.97899356802076e-14 19.0844785336537 18.1328182188905;-7e-06 -1.99772106419206e-14 19.0901741846293 18.1268217584145;-6e-06 -2.01644836319619e-14 19.0958679514802 18.120823508893;-5e-06 -2.03517546318485e-14 19.1015598336445 18.1148234709178;-4e-06 -2.05390236230974e-14 19.1072498305604 18.1088216450813;-3e-06 -2.07262905872259e-14 19.1129379416664 18.1028180319757;-2e-06 -2.09135555057516e-14 19.118624166401 18.0968126321936;-1e-06 -2.11008183601921e-14 19.1243085042031 18.0908054463277]  x5=2.82770783497871e-05  V1=ones(3,3)  V2=ones(3,3)  I1=ones(3,3)  I2=ones(3,3)  nHarmo=1  Measurements=None  Decoupling=off  VsMag0=0  VrMag0=0  VsAngle0=0  VrAngle0=0  IsMag0=0  IrMag0=0  IsAngle0=0  IrAngle0=0
      settings: LibrarySourceBlock=sps_lib/Power Grid Elements/Distributed Parameters Line
  Loading : DisplayBlock  LabelPosition=Hide  Transparency=1
  Loading_ : DisplayBlock  LabelPosition=Hide  Transparency=1
  Main Transfromer  Loading : Subsystem
  Maize mill : Subsystem
  Maize mill apparent power : MATLAB Function  TreatAsAtomicUnit=on
  Maize mill pf_ : Scope
  Maize mill profile : FromSpreadsheet  FileName=C:\Users\Baymax\Desktop\Mr.Usamah\Profiles\granular\h_pf\interpolated_maize_mill_hpf_profile.xlsx  SheetName=profile  Range=A3:C2002
  Maize milll output : Scope  NumInputPorts=2
  Miaze mill pf : MATLAB Function  TreatAsAtomicUnit=on
  Milk machine pf : Scope
  Milk machine profile : FromSpreadsheet  FileName=C:\Users\Baymax\Desktop\Mr.Usamah\Profiles\granular\h_pf\interpolated_milk_processing_plant_hpf_profile.xlsx  SheetName=profile  Range=A2:C2002
  Milk processing machine output : Scope  NumInputPorts=2
  Milk processing plant : Subsystem
  Milking machine apparent  power : MATLAB Function  TreatAsAtomicUnit=on
  Milking machine pf : MATLAB Function  TreatAsAtomicUnit=on
  Powerfactor : Display
  Single phase _loads_ Loading : Subsystem
  Solar Power : Scope  NumInputPorts=2
  Solar infeed Apparent Power : Scope
  Solar infeed Apparent power : MATLAB Function  TreatAsAtomicUnit=on
  Solar infeed pf : Scope
  Solar infeed power : Subsystem
  Solar supply power factor : MATLAB Function  TreatAsAtomicUnit=on
  System Power Factor Variations : Scope
  System Total Load : Scope
  System power factor : MATLAB Function  TreatAsAtomicUnit=on
  Terminator{,1..3} (4 alike) : Terminator
  Three phase Loads Apparent power : Scope  NumInputPorts=3
  Three-Phase Source1 : spsThreePhaseSourceLib/Three-Phase Source  InternalConnection=Yg  VoltagePhases=off  Voltage=400  PhaseAngle=0  Voltage_phases=[25e3 25e3 25e3]/sqrt(3)  PhaseAngles_phases=[0 -120 +120]  Frequency=50  NonIdealSource=off  SpecifyImpedance=off  Resistance=1e-6  Inductance=1e-6  ShortCircuitLevel=100e6  BaseVoltage=400  XRratio=7  BusType=swing  Pref=0  Qref=0  Prefabc=[10e3, 10e3, 10e3]  Qrefabc=[0, 0, 0]  Qmin=-inf  Qmax=inf
  Total Active Power : Display
  Total Reactive Power : Display
  Total active power : MATLAB Function  TreatAsAtomicUnit=on
  Total reactive power : MATLAB Function  TreatAsAtomicUnit=on
  Total system active power : Scope
  Total system apparent power : MATLAB Function  TreatAsAtomicUnit=on
  Total system reactive power : Scope
  Transformer loading : Scope  NumInputPorts=2
  V1,I1 : spsThreePhaseVIMeasurementLib/Three-Phase V-I Measurement  VoltageMeasurement=phase-to-ground  SetLabelV=on  LabelV=V1  Vpu=off  VpuLL=off  CurrentMeasurement=yes  SetLabelI=on  LabelI=I1  Ipu=off  Pbase=100e6  Vbase=500e3  OutputType=Complex  PhasorSimulation=off  PSBequivalent=0
  V2,I2 : spsThreePhaseVIMeasurementLib/Three-Phase V-I Measurement  VoltageMeasurement=phase-to-ground  SetLabelV=on  LabelV=V2  Vpu=off  VpuLL=off  CurrentMeasurement=yes  SetLabelI=on  LabelI=I2  Ipu=off  Pbase=100e6  Vbase=500e3  OutputType=Complex  PhasorSimulation=off  PSBequivalent=0
  V3,I3 : spsThreePhaseVIMeasurementLib/Three-Phase V-I Measurement  VoltageMeasurement=phase-to-ground  SetLabelV=on  LabelV=V3  Vpu=off  VpuLL=off  CurrentMeasurement=yes  SetLabelI=on  LabelI=I3  Ipu=off  Pbase=100e6  Vbase=500e3  OutputType=Complex  PhasorSimulation=off  PSBequivalent=0
  V4,I4 : spsThreePhaseVIMeasurementLib/Three-Phase V-I Measurement  VoltageMeasurement=phase-to-ground  SetLabelV=on  LabelV=V4  Vpu=off  VpuLL=off  CurrentMeasurement=yes  SetLabelI=on  LabelI=I4  Ipu=off  Pbase=100e6  Vbase=500e3  OutputType=Complex  PhasorSimulation=off  PSBequivalent=0
  V5,I5 : spsThreePhaseVIMeasurementLib/Three-Phase V-I Measurement  VoltageMeasurement=phase-to-ground  SetLabelV=on  LabelV=V5  Vpu=off  VpuLL=off  CurrentMeasurement=yes  SetLabelI=on  LabelI=I5  Ipu=off  Pbase=100e6  Vbase=500e3  OutputType=Complex  PhasorSimulation=off  PSBequivalent=0
  V6,I6 : spsThreePhaseVIMeasurementLib/Three-Phase V-I Measurement  VoltageMeasurement=phase-to-ground  SetLabelV=on  LabelV=V6  Vpu=off  VpuLL=off  CurrentMeasurement=yes  SetLabelI=on  LabelI=I6  Ipu=off  Pbase=100e6  Vbase=500e3  OutputType=Complex  PhasorSimulation=off  PSBequivalent=0
  Vin,Iin : spsThreePhaseVIMeasurementLib/Three-Phase V-I Measurement  VoltageMeasurement=phase-to-ground  SetLabelV=on  LabelV=Vin  Vpu=off  VpuLL=off  CurrentMeasurement=yes  SetLabelI=on  LabelI=Iin  Ipu=off  Pbase=100e6  Vbase=500e3  OutputType=Complex  PhasorSimulation=off  PSBequivalent=0
  Volltage drops : Scope  NumInputPorts=4
  Water Pump : Subsystem
  Water pump Apparent Power : MATLAB Function  TreatAsAtomicUnit=on
  Water pump output : Scope  NumInputPorts=2
  Water pump pf : Scope
  Water pump power factor : MATLAB Function  TreatAsAtomicUnit=on
  Water pump profile : FromSpreadsheet  FileName=C:\Users\Baymax\Desktop\Mr.Usamah\Profiles\granular\h_pf\interpolated_water_pump_hpf_profile.xlsx  SheetName=profile  Range=A2:C2002
  V_Input_A : PMIOPort  Side=Left
  V_Input_B : PMIOPort  Port=2  Side=Left
  V_Input_C : PMIOPort  Port=3  Side=Left
  Transformer _loading : Outport
  Solar infeed parameters : Outport  Port=2
  Feeder model parameters : Outport  Port=3
  Feeder voltage drop data : Outport  Port=4
  wires:
  [P4] -> Domestic loads pf/1(Total_P)
  Domestic_loads/1(S) -> [Dom_s], Total system apparent power/1(S1)
  [P4] -> Total active power/1(P1)
  [Q4] -> Total reactive power/4(Q4)
  [Dom_RP] -> Domestic /Residential loads(0.23kV)/2(Q)
  Domestic loads/1 -> [Dom_AP]
  Domestic loads/2 -> [Dom_RP]
  Domestic /Residential loads(0.23kV)/1(P_seq_v) -> Terminator3/1
  Main Transfromer  Loading/1(t1_loading) -> Gain2/1
  Water pump profile/2 -> [Water_RP]
  Domestic /Residential loads(0.23kV)/3(Qout) -> [Q4]
  [Vin] -> Filter13/1(Signal_in)
  [Q1] -> Maize mill apparent power/2(Q)
  Gain2/1 -> Transformer loading/1, [T1_L]  "Trf_1 loading"
  [T2_L] -> Bus Creator/2
  [V1] -> Filter1/1(Signal_in)
  [V5] -> Filter11/1(Signal_in)
  L4 drop/1(Voltage_drop) -> Average voltage drop/1(a), [Vdrop_L4], Volltage drops/4  "L4 drop"
  [P1] -> Maize mill apparent power/1(P)
  [P3] -> Water pump Apparent Power/1(P)
  Water Pump/1(P_seq_v) -> Terminator2/1
  Filter3/1(F_Signal_out) -> L2 drop/1(Vabc_start)
  Milk processing plant/2(Pout) -> [P2]
  [Water_AP] -> Water Pump/1(P)
  Filter6/1(F_Signal_out) -> Single phase _loads_ Loading/2(Vabc_out)
  [Iin] -> Filter14/1(Signal_in)
  [Total_P] -> System power factor/1(Total_P)
  [V3] -> Filter8/1(Signal_in)
  [water_s] -> Water pump power factor/2(Total_S)
  Total active power/1(p_total) -> [Total_P], Total Active Power/1, Total system active power/1  "Feeder active power loading"
  [V4] -> Filter10/1(Signal_in)
  System power factor/1(pf) -> [sys_pf], System Power Factor Variations/1, Powerfactor/1  "System pf"
  [Vdrop_L2] -> Bus Creator3/3
  [Milk_AP] -> Milk processing plant/1(P)
  Bus Creator3/1 -> Feeder voltage drop data/1
  Filter4/1(F_Signal_out) -> Main Transfromer  Loading/2(Vabc_out)
  Filter7/1(F_Signal_out) -> Single phase _loads_ Loading/3(Iabc_out)
  [Water_RP] -> Water Pump/2(Q)
  [Total_S] -> System power factor/2(Total_S)
  [P3] -> Total active power/4(P4)
  [P3] -> Water pump output/1
  Milk processing plant/3(Qout) -> [Q2]
  Gain3/1 -> Transformer loading/2, [T2_L]  "Trf_2 loading"
  Gain4/1 -> Solar infeed power/2(Iin)
  Filter8/1(F_Signal_out) -> L2 drop/2(Vabc_end)
  L1 drop/1(Voltage_drop) -> Average voltage drop/4(d), [Vdrop_L1], Volltage drops/1  "L1 drop"
  Bus Creator2/1 -> Feeder model parameters/1
  [Q3] -> Water pump Apparent Power/2(Q)
  Milking machine apparent  power/1(S) -> [milk_s], Three phase Loads Apparent power/2, Total system apparent power/3(S3)
  Solar infeed power/2(Inv_R) -> [INV_R], Solar Power/2, Solar infeed Apparent power/2(Q)
  Total system apparent power/1(s_total) -> [Total_S], Display2/1, System Total Load/1  "Total system apparent loading"
  [Maize_RP] -> Maize mill/2(Q)
  Maize mill/3(Qout) -> [Q1]
  [V6] -> Filter12/1(Signal_in)
  Milking machine pf/1(pf) -> Milk machine pf/1, Computed pf_/1
  [INV_pf] -> Bus Creator1/1
  [Maize_AP] -> Maize mill/1(P)
  Constant/1 -> Main Transfromer  Loading/1(Rating)
  Water Pump/3(Qout) -> [Q3]
  [Vdrop_L4] -> Bus Creator3/5
  Milk processing plant/1(P_seq_v) -> Terminator1/1
  Filter13/1(F_Signal_out) -> Gain1/1
  [P1] -> Miaze mill pf/1(Total_P)
  [P2] -> Milking machine apparent  power/1(P)
  Bus Creator/1 -> Transformer _loading/1
  Maize mill apparent power/1(S) -> Total system apparent power/4(S4), Three phase Loads Apparent power/3, [mill_s]
  Maize mill profile/2 -> [Maize_RP]
  [INV_A] -> Bus Creator1/3
  Milk machine profile/2 -> [Milk_RP]
  [V1] -> Filter4/1(Signal_in)
  Filter1/1(F_Signal_out) -> L1 drop/1(Vabc_start)
  [P3] -> Water pump power factor/1(Total_P)
  [Q1] -> Total reactive power/3(Q3)
  [mill_s] -> Miaze mill pf/2(Total_S)
  [Q1] -> Maize milll output/2
  Filter10/1(F_Signal_out) -> L3 drop/2(Vabc_end)
  [Q3] -> Water pump output/2
  Constant3/1 -> L4 drop/3(Vph_ph_norm)
  [P2] -> Total active power/3(P3)
  [T1_L] -> Bus Creator/1
  Filter11/1(F_Signal_out) -> L4 drop/1(Vabc_start)
  Average voltage drop/1(avg) -> [Vdrop], Avg voltage drop/1  "Average vdrop"
  [V2] -> Filter3/1(Signal_in)
  L3 drop/1(Voltage_drop) -> Average voltage drop/2(b), [Vdrop_L3], Volltage drops/3  "L3 drop"
  Constant1/1 -> Single phase _loads_ Loading/1(Rating)
  Constant2/1 -> L1 drop/3(Vph_ph_norm), L2 drop/3(Vph_ph_norm), L3 drop/3(Vph_ph_norm)
  Maize mill profile/1 -> [Maize_AP]
  [Total_Q] -> Bus Creator2/2
  Domestic loads pf/1(pf) -> Domestic loads pf_/1, Computed pf____/1
  Single phase _loads_ Loading/1(pload) -> Gain3/1
  [INV_S] -> Bus Creator1/2
  Water pump power factor/1(pf) -> Water pump pf/1, Computed pf/1
  Domestic /Residential loads(0.23kV)/2(Pout) -> [P4]
  [Q2] -> Milk processing machine output/2
  Total reactive power/1(q_total) -> Total Reactive Power/1, Total system reactive power/1, [Total_Q]  "Feeder reactive power loading"
  [Q3] -> Total reactive power/1(Q1)
  Solar infeed power/1(Inv_A) -> [INV_A], Solar Power/1, Solar supply power factor/1(Total_P), Solar infeed Apparent power/1(P)  "PV active power"
  Solar infeed Apparent power/1(S) -> [INV_S], Solar infeed Apparent Power/1, Solar supply power factor/2(Total_S)  "Solar apparent power supply"
  Solar supply power factor/1(pf) -> [INV_pf], Solar infeed pf/1  "Solar infeed pf"
  [I5] -> Filter7/1(Signal_in)
  [V3] -> Filter9/1(Signal_in)
  Filter12/1(F_Signal_out) -> L4 drop/2(Vabc_end)
  [Dom_s] -> Domestic loads pf/2(Total_S)
  Filter5/1(F_Signal_out) -> Main Transfromer  Loading/3(Iabc_out)
  Bus Creator1/1 -> Solar infeed parameters/1
  Water Pump/2(Pout) -> [P3]
  L2 drop/1(Voltage_drop) -> Average voltage drop/3(c), [Vdrop_L2], Volltage drops/2  "L2 drop"
  [P1] -> Maize milll output/1
  Miaze mill pf/1(pf) -> Maize mill pf_/1, Computed pf__/1
  [Milk_RP] -> Milk processing plant/2(Q)
  [P2] -> Milking machine pf/1(Total_P)
  [I1] -> Filter5/1(Signal_in)
  Filter9/1(F_Signal_out) -> L3 drop/1(Vabc_start)
  [Q2] -> Total reactive power/2(Q2)
  [Vdrop_L3] -> Bus Creator3/4
  Maize mill/1(P_seq_v) -> Terminator/1
  [V2] -> Filter2/1(Signal_in)
  [Total_P] -> Bus Creator2/1
  [Q4] -> Domestic_loads/2(Q)
  Filter14/1(F_Signal_out) -> Gain4/1
  Milk machine profile/1 -> [Milk_AP]
  Water pump profile/1 -> [Water_AP]
  [P2] -> Milk processing machine output/1
  [V5] -> Filter6/1(Signal_in)
  [P1] -> Total active power/2(P2)
  [Dom_AP] -> Domestic /Residential loads(0.23kV)/1(P)
  Gain1/1 -> Solar infeed power/1(Vin)
  Water pump Apparent Power/1(S) -> Three phase Loads Apparent power/1, [water_s], Total system apparent power/2(S2)
  [milk_s] -> Milking machine pf/2(Total_S)
  [sys_pf] -> Bus Creator2/4
  [Vdrop_L1] -> Bus Creator3/2
  [Vdrop] -> Bus Creator3/1
  [Total_S] -> Bus Creator2/3
  [Q2] -> Milking machine apparent  power/2(Q)
  [P4] -> Domestic_loads/1(P)
  Filter2/1(F_Signal_out) -> L1 drop/2(Vabc_end)
  Maize mill/2(Pout) -> [P1]
  [P4] -> Domestic loads_output/1
  [Q4] -> Domestic loads_output/2
  connections:
  "11kV/400V "/RConn1 -- Vin,Iin/RConn1 -- Three-Phase Source1/RConn1 -- V1,I1/LConn1
  "11kV/400V "/RConn3 -- Vin,Iin/RConn3 -- Three-Phase Source1/RConn3 -- V1,I1/LConn3
  L3_5km/LConn2 -- Milk processing plant/LConn2 -- V3,I3/RConn2 -- "400/230V-10kVA "/LConn2
  "11kV/400V "/RConn2 -- Vin,Iin/RConn2 -- Three-Phase Source1/RConn2 -- V1,I1/LConn2
  L3_5km/LConn1 -- "400/230V-10kVA "/LConn1 -- Milk processing plant/LConn1 -- V3,I3/RConn1
  Milk processing plant/LConn3 -- "400/230V-10kVA "/LConn3 -- V3,I3/RConn3 -- L3_5km/LConn3
  L2_3km/LConn2 -- Maize mill/LConn2 -- V2,I2/RConn2
  L2_3km/LConn3 -- Maize mill/LConn3 -- V2,I2/RConn3
  L2_3km/LConn1 -- Maize mill/LConn1 -- V2,I2/RConn1
  V6,I6/RConn2 -- Domestic /Residential loads(0.23kV)/LConn2
  L3_5km/RConn2 -- V4,I4/LConn2
  V4,I4/RConn3 -- Water Pump/LConn3
  V5,I5/LConn1 -- "400/230V-10kVA "/RConn1
  V4,I4/RConn2 -- Water Pump/LConn2
  V_Input_C/RConn1 -- Vin,Iin/LConn3
  "400/230V-10kVA "/RConn3 -- V5,I5/LConn3
  L2_3km/RConn3 -- V3,I3/LConn3
  L4_5km/LConn3 -- V5,I5/RConn1
  L3_5km/RConn1 -- V4,I4/LConn1
  L2_3km/RConn1 -- V3,I3/LConn1
  L4_5km/RConn2 -- V6,I6/LConn2
  L2_3km/RConn2 -- V3,I3/LConn2
  L1_10km/RConn2 -- V2,I2/LConn2
  L1_10km/RConn1 -- V2,I2/LConn1
  11kV Main supply/RConn2 -- "11kV/400V "/LConn2
  L1_10km/LConn2 -- V1,I1/RConn2
  V6,I6/RConn3 -- Domestic /Residential loads(0.23kV)/LConn3
  L4_5km/LConn1 -- V5,I5/RConn3
  V5,I5/LConn2 -- "400/230V-10kVA "/RConn2
  L4_5km/LConn2 -- V5,I5/RConn2
  L3_5km/RConn3 -- V4,I4/LConn3
  V4,I4/RConn1 -- Water Pump/LConn1
  L4_5km/RConn3 -- V6,I6/LConn1
  L4_5km/RConn1 -- V6,I6/LConn3
  11kV Main supply/RConn1 -- "11kV/400V "/LConn1
  V_Input_B/RConn1 -- Vin,Iin/LConn2
  11kV Main supply/RConn3 -- "11kV/400V "/LConn3
  L1_10km/RConn3 -- V2,I2/LConn3
  L1_10km/LConn1 -- V1,I1/RConn1
  L1_10km/LConn3 -- V1,I1/RConn3
  V_Input_A/RConn1 -- Vin,Iin/LConn1
  Domestic /Residential loads(0.23kV)/LConn1 -- V6,I6/RConn1
